simulink model "problem7"  (R2020a)
settings: Solver=VariableStepAuto  StartTime=0.0  StopTime=10.0  RelTol=1e-3
libraries: simulink x1
settings Model: Creator=Riyansh  LastModifiedBy=Riyansh

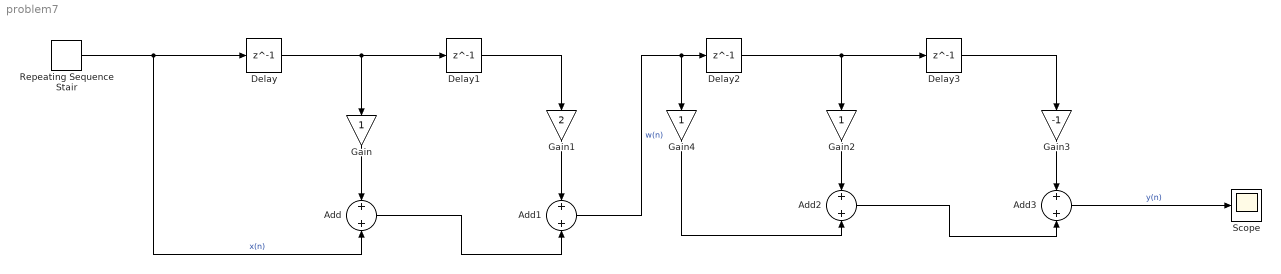
== system problem7 ==
  Add{,1..3} (4 alike) : Sum
  Delay{,1..3} (4 alike) : Delay  DelayLength=1
  Gain : Gain
  Gain1 : Gain  Gain=2
  Gain2 : Gain
  Gain3 : Gain  Gain=-1
  Gain4 : Gain
  Repeating Sequence Stair : simulink/Sources/Repeating Sequence Stair  OutValues=[3 1 4 2 1].'  tsamp=-1  OutMin=[]  OutMax=[]  OutDataTypeStr=double  OutputDataTypeScalingMode=double  OutDataType=fixdt(0,8)  ConRadixGroup=Best Precision: Vector-wise  OutScaling=2^-12
  Scope : Scope
  wires:
  Add3/1 -> Scope/1  "y(n)"
  Gain2/1 -> Add2/1
  Gain/1 -> Add/1
  Gain1/1 -> Add1/1
  Delay/1 -> Delay1/1, Gain/1
  Gain3/1 -> Add3/1
  Repeating Sequence Stair/1 -> Add/2, Delay/1  "x(n)"
  Add2/1 -> Add3/2
  Delay2/1 -> Delay3/1, Gain2/1
  Gain4/1 -> Add2/2
  Delay1/1 -> Gain1/1
  Add1/1 -> Delay2/1, Gain4/1  "w(n)"
  Delay3/1 -> Gain3/1
  Add/1 -> Add1/2
